simulink model "Cartesian_Regulation_ROS"  (R2022b)
settings: Solver=FixedStepAuto  StartTime=0.0  StopTime=inf  FixedStep=0.02  MaxStep=0.1  RelTol=1e-3
undefined symbols (not defined in the file): unicycle, X, x_f, Y, y_f
libraries: robotlib x3, simulink_extras x1
settings Model: Creator=hp 2021  LastModifiedBy=Musta
settings OptimizationCC: EnhancedBackFolding=on  PassReuseOutputArgsAs=Individual arguments  ZeroExternalMemoryAtStartup=off  ZeroInternalMemoryAtStartup=off  MaxStackSize=64  OptimizeBlockOrder=speed  DifferentSizesBufferReuse=on  OptimizationCustomize=off  EfficientTunableParamExpr=on
settings DebuggingCC: ParameterTunabilityLossMsg=error
settings HardwareCC: ProdBitPerPointer=32  ProdBitPerSizeT=32  ProdBitPerPtrDiffT=32  ProdLargestAtomicFloat=None  ProdIntDivRoundTo=Undefined  ProdEndianess=Unspecified  ProdWordSize=32  ProdHWDeviceType=Generic->Unspecified (assume 32-bit Generic)
settings ModelReferenceCC: EnableRefExpFcnMdlSchedulingChecks=on
settings SFSimCC: MATLABDynamicMemAlloc=off
settings RTWCC: Description=Embedded Coder  SystemTargetFile=ert.tlc  HardwareBoard=Robot Operating System (ROS)  TLCOptions="-aInlineSetEventsForThisBaseRateFcn=TLC_FALSE -aSuppressMultiTaskScheduler=TLC_FALSE  -aRateBasedStepFcn=0"  TemplateMakefile=ert_default_tmf  Toolchain=Catkin  TargetLang=C++
settings CodeAppCC: ForceParamTrailComments=on  IgnoreCustomStorageClasses=off  OperatorAnnotations=on  SimulinkDataObjDesc=on  SFDataObjDesc=on  InsertBlockDesc=on

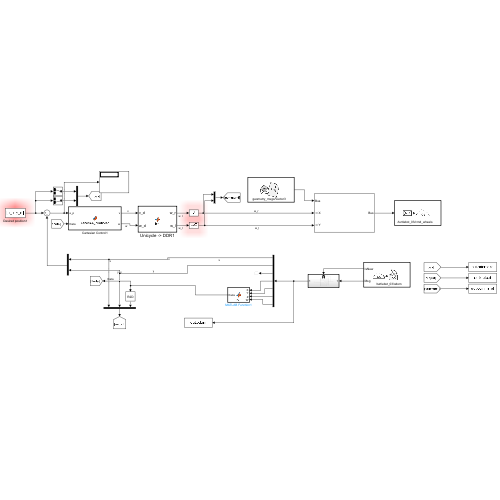
[thumbnail: Simulink's stored preview of the top-level diagram]
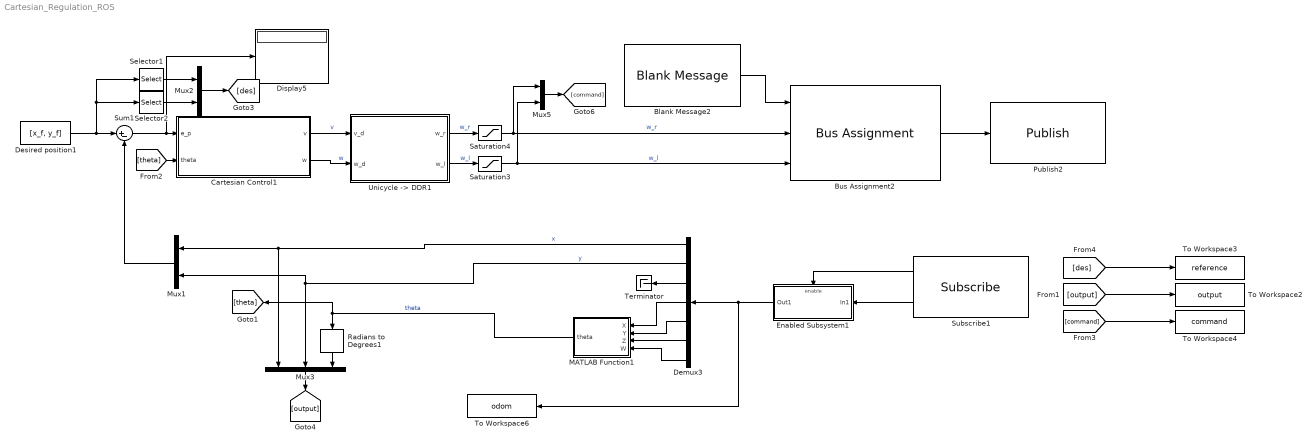
== system Cartesian_Regulation_ROS ==
  Blank Message2 : robotlib/Blank Message  messageClass=Message  entityType=geometry_msgs/Vector3  messageType=geometry_msgs/Vector3  SampleTime=0.02  legacyBusStruct=off
      settings: LibrarySourceBlock=roslib/ROS/Blank Message
  Bus Assignment2 : BusAssignment  AssignedSignals=X,Y
  Cartesian Control1 : MATLAB Function  TreatAsAtomicUnit=on
  Demux3 : Demux  Outputs=7
  Desired position1 : Constant  Value=[x_f, y_f]
  Display5 : Display
  Enabled Subsystem1 : Subsystem  TreatAsAtomicUnit=on
  MATLAB Function1 : MATLAB Function  TreatAsAtomicUnit=on
  Mux1 : Mux  Inputs=2
  Mux2 : Mux  Inputs=2
  Mux3 : Mux  Inputs=3
  Mux5 : Mux  Inputs=2
  Publish2 : robotlib/Publish  topicSource=Select from ROS network  topic=/turtlebot_03/cmd_wheels  messageType=geometry_msgs/Vector3  legacyBusStruct=off  messageQueueLength=1
      settings: LibrarySourceBlock=roslib/ROS/Publish
  Radians to Degrees1 : simulink_extras/Transformations/Radians to Degrees
  Saturation3 : Saturate  UpperLimit=unicycle.omegaWheelMax  LowerLimit=unicycle.omegaWheelMin
  Saturation4 : Saturate  UpperLimit=unicycle.omegaWheelMax  LowerLimit=unicycle.omegaWheelMin
  Selector1 : Selector  InputPortWidth=2  IndexOptions=Index vector (dialog)  Indices=1  OutputSizes=1
  Selector2 : Selector  InputPortWidth=2  IndexOptions=Index vector (dialog)  Indices=2  OutputSizes=1
  Subscribe1 : robotlib/Subscribe  topicSource=Select from ROS network  topic=/turtlebot_03/odom  messageType=nav_msgs/Odometry  SampleTime=0.02  legacyBusStruct=off  messageQueueLength=1
      settings: LibrarySourceBlock=roslib/ROS/Subscribe
  Sum1 : Sum  Inputs=|+-
  Terminator : Terminator
  To Workspace2 : ToWorkspace  VariableName=output  SaveFormat=Structure With Time  SampleTime=-1
  To Workspace3 : ToWorkspace  VariableName=reference  SaveFormat=Structure With Time  SampleTime=-1
  To Workspace4 : ToWorkspace  VariableName=command  SaveFormat=Structure With Time  SampleTime=-1
  To Workspace6 : ToWorkspace  VariableName=odom  SaveFormat=Structure With Time  SampleTime=-1
  "Unicycle -> DDR1" : MATLAB Function  TreatAsAtomicUnit=on
  wires:
  [command] -> To Workspace4/1
  [output] -> To Workspace2/1
  [des] -> To Workspace3/1
  Mux1/1 -> Sum1/2
  Saturation4/1 -> Bus Assignment2/2, Mux5/1  "w_r"
  MATLAB Function1/1(theta) -> [theta], Radians to Degrees1/1  "theta"
  [theta] -> Cartesian Control1/2(theta)
  Radians to Degrees1/1 -> Mux3/3
  Sum1/1 -> Display5/1, Cartesian Control1/1(e_p)
  Selector1/1 -> Mux2/1
  Desired position1/1 -> Sum1/1, Selector2/1, Selector1/1
  Mux2/1 -> [des]
  Mux3/1 -> [output]
  Selector2/1 -> Mux2/2
  Mux5/1 -> [command]
  Blank Message2/1 -> Bus Assignment2/1
  Cartesian Control1/1(v) -> "Unicycle -> DDR1"/1(v_d)  "v"
  Bus Assignment2/1 -> Publish2/1
  "Unicycle -> DDR1"/2(w_l) -> Saturation3/1  "w_l"
  "Unicycle -> DDR1"/1(w_r) -> Saturation4/1  "w_r"
  Saturation3/1 -> Bus Assignment2/3, Mux5/2  "w_l"
  Cartesian Control1/2(w) -> "Unicycle -> DDR1"/2(w_d)  "w"
  Demux3/3 -> Terminator/1
  Subscribe1/2 -> Enabled Subsystem1/1(In1)
  Demux3/1 -> Mux3/1, Mux1/1  "x"
  Subscribe1/1 -> Enabled Subsystem1/Enable
  Enabled Subsystem1/1(Out1) -> Demux3/1, To Workspace6/1
  Demux3/2 -> Mux1/2, Mux3/2  "y"
  Demux3/6 -> MATLAB Function1/3(Z)
  Demux3/5 -> MATLAB Function1/2(Y)
  Demux3/7 -> MATLAB Function1/4(W)
  Demux3/4 -> MATLAB Function1/1(X)

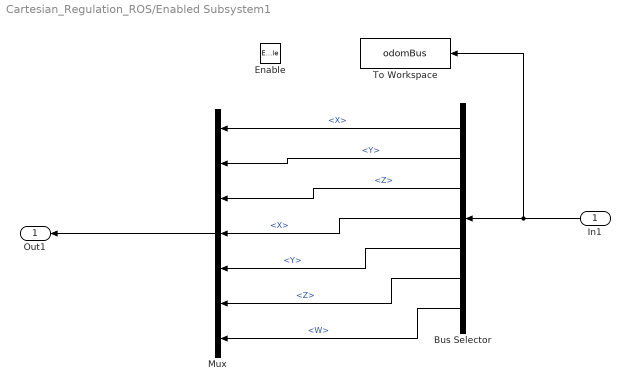
== system Cartesian_Regulation_ROS/Enabled Subsystem1 ==
  In1 : Inport
  Enable : EnablePort
  Bus Selector : BusSelector  OutputSignals=Pose.Pose.Position.X,Pose.Pose.Position.Y,Pose.Pose.Position.Z,Pose.Pose.Orientation.X,Pose.Pose.Orientation.Y,Pose.Pose.Orientation.Z,Pose.Pose.Orientation.W
  Mux : Mux  Inputs=7
  To Workspace : ToWorkspace  VariableName=odomBus  SaveFormat=Timeseries  SampleTime=-1
  Out1 : Outport
  wires:
  Mux/1 -> Out1/1
  Bus Selector/1 -> Mux/1  "<X>"
  Bus Selector/2 -> Mux/2  "<Y>"
  In1/1 -> To Workspace/1, Bus Selector/1
  Bus Selector/3 -> Mux/3  "<Z>"
  Bus Selector/4 -> Mux/4  "<X>"
  Bus Selector/5 -> Mux/5  "<Y>"
  Bus Selector/6 -> Mux/6  "<Z>"
  Bus Selector/7 -> Mux/7  "<W>"

== matlab function Cartesian_Regulation_ROS/Cartesian Control1 ==
  data: v output; w output; e_p input; theta input
function [v,w] = cartesian_controller(e_p, theta)

    %     %#codegen
%     coder.extrinsic('evalin')
%     K_v = 0;                  % Needed in order to set variable class correctly
%     K_w = 0;                  % Needed in order to set variable class correctly
%     K_v = evalin('base','K_v'); % Read value from workspace
%     K_w = evalin('base','K_w'); % Read value from workspace
% 
%     v = K_v * (e_p(1)*cos(theta) + e_p(2)*sin(theta));
%     w = K_w * (atan2(e_p(2),e_p(1)) - theta);

        %#codegen
    coder.extrinsic('evalin')
    K_v = 0;                  % Needed in order to set variable class correctly
    K_w = 0;                  % Needed in order to set variable class correctly
    K_v = evalin('base','K_v'); % Read value from workspace
    K_w = evalin('base','K_w'); % Read value from workspace

    v = K_v * (e_p(1)*cos(theta) + e_p(2)*sin(theta));
    p = atan2(e_p(2),e_p(1)) - theta;
    % Count the number of turns around full circle
    num_turns = floor(p/(2*pi));
    % Adjust p to remove any full circle turns
    theta_adj = p - num_turns*(2*pi);
    w = K_w * (theta_adj);

end

== matlab function Cartesian_Regulation_ROS/MATLAB Function1 ==
  data: X input; theta output; Y input; Z input; W input
function theta = fcn(X, Y, Z, W)

    q_x = X;
    q_y = Y;
    q_z = Z;
    q_w = W;
    
    q = cat(2,q_x,q_y,q_z,q_w); 
    eulZYX = quat2eul(q,'ZYX');
    theta = eulZYX(:,3);
    
end

== matlab function Cartesian_Regulation_ROS/Unicycle -> DDR1 ==
  data: v_d input; w_r output; w_d input; w_l output
function [w_r, w_l] = fcn(v_d, w_d)

    %#codegen
    coder.extrinsic('evalin')
    d = 0;                  % Needed in order to set variable class correctly
    r = 0;                  % Needed in order to set variable class correctly
    d = evalin('base','unicycle.d'); % Read value from workspace
    r = evalin('base','unicycle.r'); % Read value from workspace

    w_r = ((2 * v_d) + (w_d * d)) / (2 * r);
    w_l = ((2 * v_d) - (w_d * d)) / (2 * r);

end
